simulink model "PAM"  (R2020a)
settings: Solver=VariableStepAuto  StartTime=0.0  StopTime=10.0  RelTol=1e-3
libraries: dspsigops x1, dspsrcs4 x1
settings Model: Creator=jeeva  LastModifiedBy=jeeva

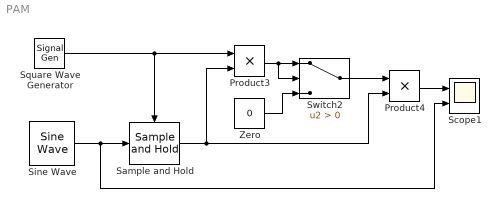
== system PAM ==
  Product3 : Product
  Product4 : Product
  Sample and Hold : dspsigops/Sample and Hold  trig=Rising edge  initCond=0  latchinput=off
  Scope1 : Scope  NumInputPorts=2
  Sine Wave : dspsrcs4/Sine Wave  Amplitude=1  Frequency=0.2  Phase=0  SampleMode=Discrete  OutComplex=Real  CompMethod=Trigonometric fcn  TableSize=Speed  SampleTime=1/1000  SamplesPerFrame=1  ResetState=Restart at time zero  OutputFrames=off  dataType=double  wordLen=16  udDataType=sfix(16)  fracBitsMode=Best precision  numFracBits=15  OutDataTypeStr=double  LastOutDataTypeStr=double
  Square Wave Generator : SignalGenerator  WaveForm=square  Frequency=5
  Switch2 : Switch  Criteria=u2 > Threshold
  Zero : Constant  Value=0  OutDataTypeStr=Inherit: Inherit via back propagation
  wires:
  Sine Wave/1 -> Sample and Hold/1, Scope1/2
  Square Wave Generator/1 -> Sample and Hold/Trigger, Product3/1
  Sample and Hold/1 -> Product4/2, Product3/2
  Zero/1 -> Switch2/3
  Product3/1 -> Switch2/2, Switch2/1
  Switch2/1 -> Product4/1
  Product4/1 -> Scope1/1
